simulink model "RLC_MODEL_SIMULINK"  (R2022b)
settings: Solver=ode4  StartTime=0.0  StopTime=10.0  FixedStep=StepSize  RelTol=1e-3
values from neighbouring files (symbols this model uses):
  C = 100e-6    (= 0.0001)    [RLC_MODEL_SCRIPT.m]
  L = 300e-1    (= 30)    [RLC_MODEL_SCRIPT.m]
  R = 240    [RLC_MODEL_SCRIPT.m]
  Um = sqrt(2)*U    [RLC_MODEL_SCRIPT.m]
  w = 2*pi*f    (= 314.159265359)    [RLC_MODEL_SCRIPT.m]
settings Model: Creator=irfan  LastModifiedBy=irfan

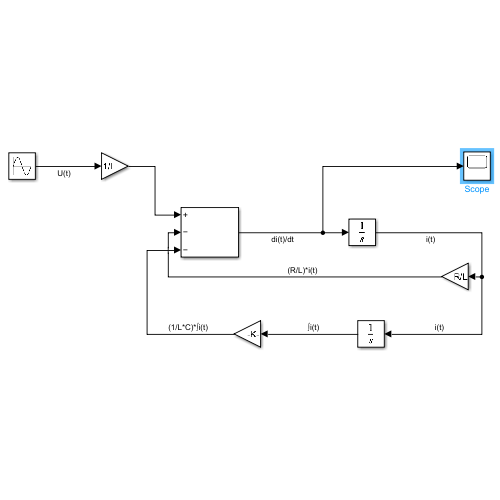
[thumbnail: Simulink's stored preview of the top-level diagram]
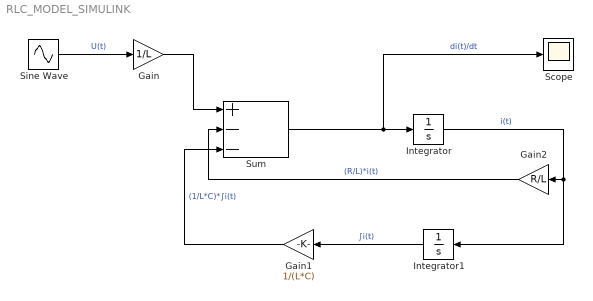
== system RLC_MODEL_SIMULINK ==
  Gain : Gain  Gain=1/L
  Gain1 : Gain  Gain=1/(L*C)
  Gain2 : Gain  Gain=R/L
  Integrator : Integrator
  Integrator1 : Integrator
  Scope : Scope
  Sine Wave : Sin  Amplitude=Um  Frequency=w  SampleTime=0
  Sum : Sum  Inputs=+--
  wires:
  Sine Wave/1 -> Gain/1  "U(t)"
  Gain/1 -> Sum/1
  Sum/1 -> Scope/1, Integrator/1  "di(t)/dt"
  Integrator/1 -> Integrator1/1, Gain2/1  "i(t)"
  Gain2/1 -> Sum/2  "(R/L)*i(t)"
  Integrator1/1 -> Gain1/1  "∫i(t)"
  Gain1/1 -> Sum/3  "(1/L*C)*∫i(t)"
